simulink model "DemoModel"  (R2018b)
settings: Solver=FixedStepAuto  StartTime=0.0  StopTime=t_final  FixedStep=dt  RelTol=1e-3
values from neighbouring files (symbols this model uses):
  dt = 1/20    (= 0.05)    [MAIN_InitializeModel.m]
  h0_m = 500    [MAIN_InitializeModel.m]
  lat0_deg = ConvertLatLonDegMinSecToDecimal(21,19,28.25)    [MAIN_InitializeModel.m]
  lon0_deg = ConvertLatLonDegMinSecToDecimal(-157,55,30.26)    [MAIN_InitializeModel.m]
libraries: aerolibfltsims x2
settings Model: Creator=Christopher  LastModifiedBy=Christopher

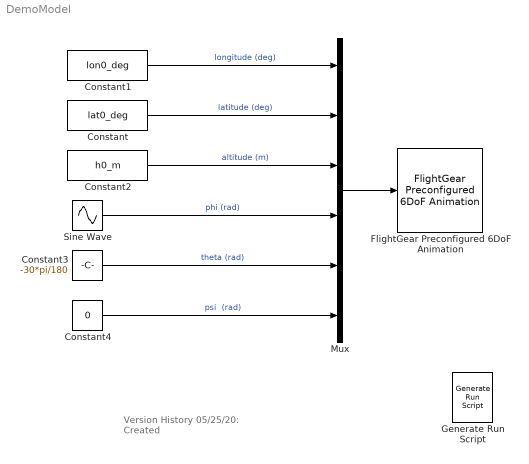
== system DemoModel ==
  note: Version History
      | 05/25/20: Created
  Constant : Constant  Value=lat0_deg
  Constant1 : Constant  Value=lon0_deg
  Constant2 : Constant  Value=h0_m
  Constant3 : Constant  Value=-30*pi/180
  Constant4 : Constant  Value=0
  FlightGear Preconfigured 6DoF Animation : aerolibfltsims/FlightGear Preconfigured 6DoF Animation  xFlightGearVersion=v2018.1  DestinationIpAddress=127.0.0.1  DestinationPort=5502  SampleTime=dt  packetVersion=24
      settings: SourceProductName=Aerospace Blockset
  Generate Run Script : aerolibfltsims/Generate Run Script  Architecture=Win64  dataFlow=Send  GeometryModelName=c172p  AirportId=KSFO  RunwayId=10L  InitialAltitude=7224  InitialHeading=113  OffsetDistance=4.72  OffsetAzimuth=0  InstallScenery=off  DisableShaders=off  OriginAddress=127.0.0.1  DestinationPort=5502  OriginPort=5505  LocalAddress=127.0.0.1  OutputFileName=runfg.bat  FlightGearBaseDirectory=C:\Program Files\FlightGear 2018.1.1
  Mux : Mux  Inputs=6
  Sine Wave : Sin  Amplitude=30*pi/180  SampleTime=0
  wires:
  Mux/1 -> FlightGear Preconfigured 6DoF Animation/1
  Constant1/1 -> Mux/1  "longitude (deg)"
  Constant/1 -> Mux/2  "latitude (deg)"
  Constant2/1 -> Mux/3  "altitude (m)"
  Sine Wave/1 -> Mux/4  "phi (rad)"
  Constant3/1 -> Mux/5  "theta (rad)"
  Constant4/1 -> Mux/6  "psi  (rad)"
